simulink model "sp1450WECSminiProject1"  (R2013a)
settings: Solver=ode45  SolverMode=SingleTasking  StartTime=0.0  StopTime=1  RelTol=1e-3
undefined symbols (not defined in the file): D1, J, Lm, Lr, Ls, P, Rr, Rs
libraries: powerlib x8, sdolib x2
settings Model: Creator=Waseem  LastModifiedBy=Sony
settings DataIOCC: SignalLoggingSaveFormat=ModelDataLogs
settings OptimizationCC: BlockReduction=off  BooleanDataType=off
settings DebuggingCC: SaveWithParameterizedLinksMsg=none  SignalResolutionControl=TryResolveAllWithWarning  SolverPrmCheckMsg=none  MultiTaskDSMMsg=warning  MultiTaskCondExecSysMsg=none  StrictBusMsg=None
settings HardwareCC: TargetUnknown=on
settings RTWCC: IncludeERTFirstTime=on

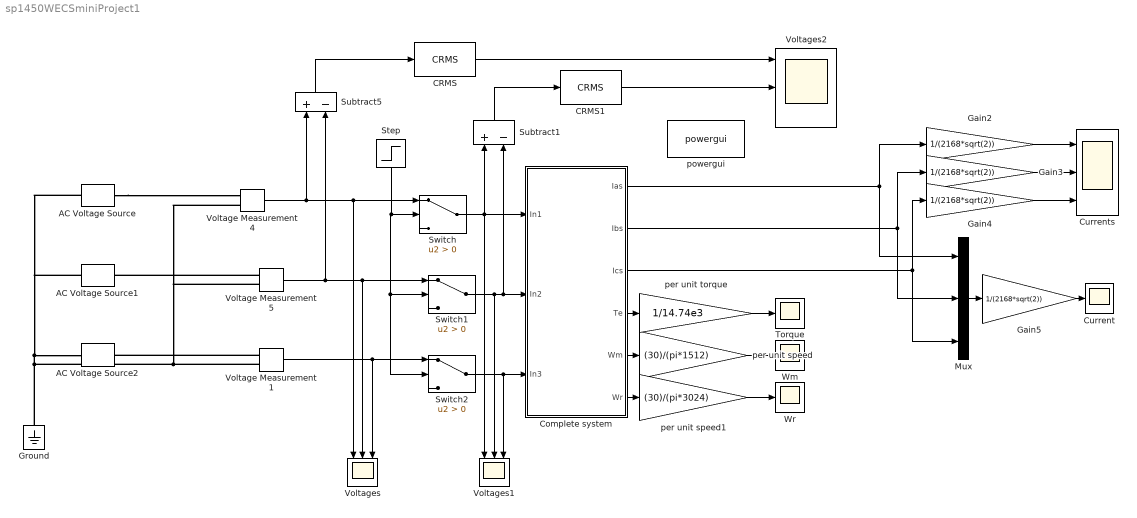
== system sp1450WECSminiProject1 ==
  AC Voltage Source : powerlib/Electrical Sources/AC Voltage Source  Amplitude=563.38264  Phase=0  Frequency=50  SampleTime=0  Measurements=None
  AC Voltage Source1 : powerlib/Electrical Sources/AC Voltage Source  Amplitude=563.38264  Phase=-120  Frequency=50  SampleTime=0  Measurements=None
  AC Voltage Source2 : powerlib/Electrical Sources/AC Voltage Source  Amplitude=563.38264  Phase=-240  Frequency=50  SampleTime=0  Measurements=None
  CRMS : sdolib/RMS Blocks/CRMS
  CRMS1 : sdolib/RMS Blocks/CRMS
  Complete system : Subsystem
  Current : Scope
  Currents : Scope  NumInputPorts=3
      settings: YMin=-5~-5~-5  YMax=5~5~5
  Gain{2..5} (4 alike) : Gain  Gain=1/(2168*sqrt(2))
  Ground : powerlib/Elements/Ground  LConnTagsString=a
  Mux : Mux  Inputs=3
  Step : Step  Time=0  SampleTime=0
  Subtract1 : Sum  Inputs=+-
  Subtract5 : Sum  Inputs=+-
  Switch : Switch  Criteria=u2 > Threshold
  Switch1 : Switch  Criteria=u2 > Threshold
  Switch2 : Switch  Criteria=u2 > Threshold
  Torque : Scope
      settings: YMin=-1.863e-05  YMax=-1.847e-05
  Voltage Measurement1 : powerlib/Measurements/Voltage Measurement  PhasorSimulation=off  OutputType=Complex  PSBequivalent=0
  Voltage Measurement4 : powerlib/Measurements/Voltage Measurement  PhasorSimulation=off  OutputType=Complex  PSBequivalent=0
  Voltage Measurement5 : powerlib/Measurements/Voltage Measurement  PhasorSimulation=off  OutputType=Complex  PSBequivalent=0
  Voltages : Scope  NumInputPorts=3
      settings: YMin=-5~-5~-5  YMax=5~5~5
  Voltages1 : Scope  NumInputPorts=3
      settings: YMin=-5~-5~-5  YMax=5~5~5
  Voltages2 : Scope  NumInputPorts=3
      settings: YMin=-5~-5~-5  YMax=5~5~5  SaveName=ScopeData2
  Wm : Scope
      settings: YMin=37.89  YMax=38.09
  Wr : Scope
      settings: YMin=37.89  YMax=38.09  SaveName=ScopeData3
  per unit speed : Gain  Gain=(30)/(pi*1512)
  per unit speed1 : Gain  Gain=(30)/(pi*3024)
  per unit torque : Gain  Gain=1/14.74e3
  powergui : powerlib/powergui  Priority=1  SimulationMode=Continuous  SolverType=Tustin  SampleTime=50e-6  frequency=50  SPID=on  DisableSnubberDevices=off  DisableRonSwitches=off  DisableVfSwitches=off  SwTol=0  Interpol=off  DisplayEquations=off  frequencyindice=50  Pbase=100e6  ErrMax=1e-4  Iterations=50  UnitsV=kV  UnitsW=MW  FunctionMessages=off  echomessages=off  HookPort=off  EnableUseOfTLC=off  x0status=blocks  RestoreLinks=warning  ResistiveCurrentMeasurement=off  Frange=[0:2:500]  Ylog=off  Xlog=on  ShowGrid=off  save=off  variable=ZData  ZoomFFT=off  StartTime=0.0  cycles=1  DisplayStyle=1  fundamental=60  FreqAxis=off  MaxFrequency=1000  frequencyindicesteady=1  RmsSteady=1  display=off  Ts=0  methode=off
  wires:
  Mux/1 -> Gain5/1
  Voltage Measurement1/1 -> Switch2/1, Voltages/3
  Voltage Measurement5/1 -> Voltages/2, Switch1/1, Subtract5/2
  Complete system/2(Ibs) -> Mux/2, Gain3/1
  Complete system/3(Ics) -> Mux/3, Gain4/1
  Complete system/1(Ias) -> Mux/1, Gain2/1
  Complete system/4(Te) -> per unit torque/1
  Complete system/5(Wm) -> per unit speed/1
  per unit speed/1 -> Wm/1
  Gain2/1 -> Currents/1
  Gain3/1 -> Currents/2
  Gain4/1 -> Currents/3
  Gain5/1 -> Current/1
  Switch/1 -> Subtract1/1, Complete system/1(In1), Voltages1/1
  Switch2/1 -> Complete system/3(In3), Voltages1/3
  Switch1/1 -> Voltages1/2, Complete system/2(In2), Subtract1/2
  Step/1 -> Switch2/2, Switch1/2, Switch/2
  Voltage Measurement4/1 -> Voltages/1, Switch/1, Subtract5/1
  CRMS/1 -> Voltages2/1
  Subtract5/1 -> CRMS/1
  CRMS1/1 -> Voltages2/2
  Subtract1/1 -> CRMS1/1
  per unit torque/1 -> Torque/1
  Complete system/6(Wr) -> per unit speed1/1
  per unit speed1/1 -> Wr/1
  connections:
  Ground/LConn1 -- AC Voltage Source1/LConn1 -- AC Voltage Source/LConn1 -- AC Voltage Source2/LConn1 -- Voltage Measurement5/LConn2 -- Voltage Measurement4/LConn2 -- Voltage Measurement1/LConn2
  AC Voltage Source/RConn1 -- Voltage Measurement4/LConn1
  Voltage Measurement5/LConn1 -- AC Voltage Source1/RConn1
  Voltage Measurement1/LConn1 -- AC Voltage Source2/RConn1

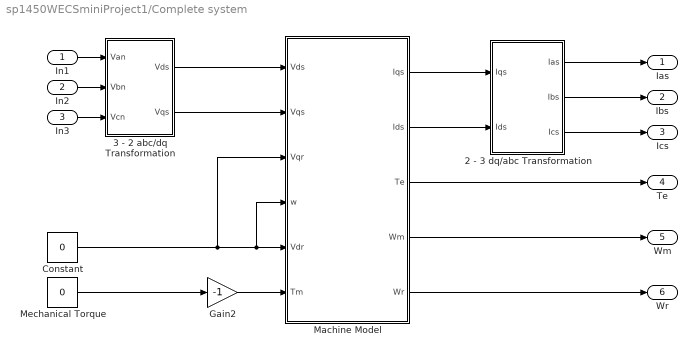
== system sp1450WECSminiProject1/Complete system ==
  In1 : Inport
  In2 : Inport  Port=2
  In3 : Inport  Port=3
  2 - 3 dq/abc Transformation : Subsystem
  3 - 2 abc/dq Transformation : Subsystem
  Constant : Constant  Value=0
  Gain2 : Gain  Gain=-1  ParamDataTypeStr=double
  Machine Model : Subsystem
  Mechanical Torque : Constant  Value=0
  Ias : Outport
  Ibs : Outport  Port=2
  Ics : Outport  Port=3
  Te : Outport  Port=4
  Wm : Outport  Port=5
  Wr : Outport  Port=6
  wires:
  2 - 3 dq/abc Transformation/2(Ibs) -> Ibs/1
  2 - 3 dq/abc Transformation/3(Ics) -> Ics/1
  2 - 3 dq/abc Transformation/1(Ias) -> Ias/1
  Constant/1 -> Machine Model/3(Vqr), Machine Model/4(w), Machine Model/5(Vdr)
  Machine Model/4(Wm) -> Wm/1
  Machine Model/1(Iqs) -> 2 - 3 dq/abc Transformation/1(Iqs)
  3 - 2 abc/dq Transformation/1(Vds) -> Machine Model/1(Vds)
  Machine Model/2(Ids) -> 2 - 3 dq/abc Transformation/2(Ids)
  3 - 2 abc/dq Transformation/2(Vqs) -> Machine Model/2("Vqs ")
  Gain2/1 -> Machine Model/6(Tm)
  Machine Model/3(Te) -> Te/1
  Mechanical Torque/1 -> Gain2/1
  In2/1 -> 3 - 2 abc/dq Transformation/2(Vbn)
  In1/1 -> 3 - 2 abc/dq Transformation/1(Van)
  In3/1 -> 3 - 2 abc/dq Transformation/3(Vcn)
  Machine Model/5(Wr) -> Wr/1

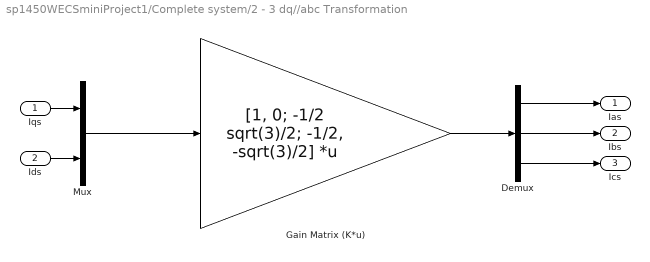
== system sp1450WECSminiProject1/Complete system/2 - 3 dq//abc Transformation ==
  Iqs : Inport
  Ids : Inport  Port=2
  Demux : Demux  Outputs=3
  Gain Matrix (K*u) : Gain  Gain=[1, 0; -1/2 sqrt(3)/2; -1/2, -sqrt(3)/2]  Multiplication=Matrix(K*u)
  Mux : Mux  Inputs=2
  Ias : Outport
  Ibs : Outport  Port=2
  Ics : Outport  Port=3
  wires:
  Mux/1 -> Gain Matrix (K*u)/1
  Gain Matrix (K*u)/1 -> Demux/1
  Demux/2 -> Ibs/1
  Demux/1 -> Ias/1
  Demux/3 -> Ics/1
  Iqs/1 -> Mux/1
  Ids/1 -> Mux/2

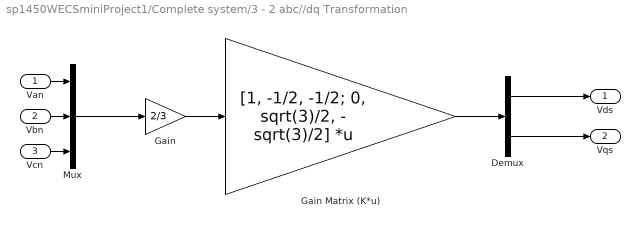
== system sp1450WECSminiProject1/Complete system/3 - 2 abc//dq Transformation ==
  Van : Inport
  Vbn : Inport  Port=2
  Vcn : Inport  Port=3
  Demux : Demux  Outputs=2
  Gain : Gain  Gain=2/3
  Gain Matrix (K*u) : Gain  Gain=[1, -1/2, -1/2; 0, sqrt(3)/2, - sqrt(3)/2]  Multiplication=Matrix(K*u)
  Mux : Mux  Inputs=3
  Vds : Outport
  Vqs : Outport  Port=2
  wires:
  Vcn/1 -> Mux/3
  Vbn/1 -> Mux/2
  Van/1 -> Mux/1
  Gain/1 -> Gain Matrix (K*u)/1
  Gain Matrix (K*u)/1 -> Demux/1
  Mux/1 -> Gain/1
  Demux/1 -> Vds/1
  Demux/2 -> Vqs/1

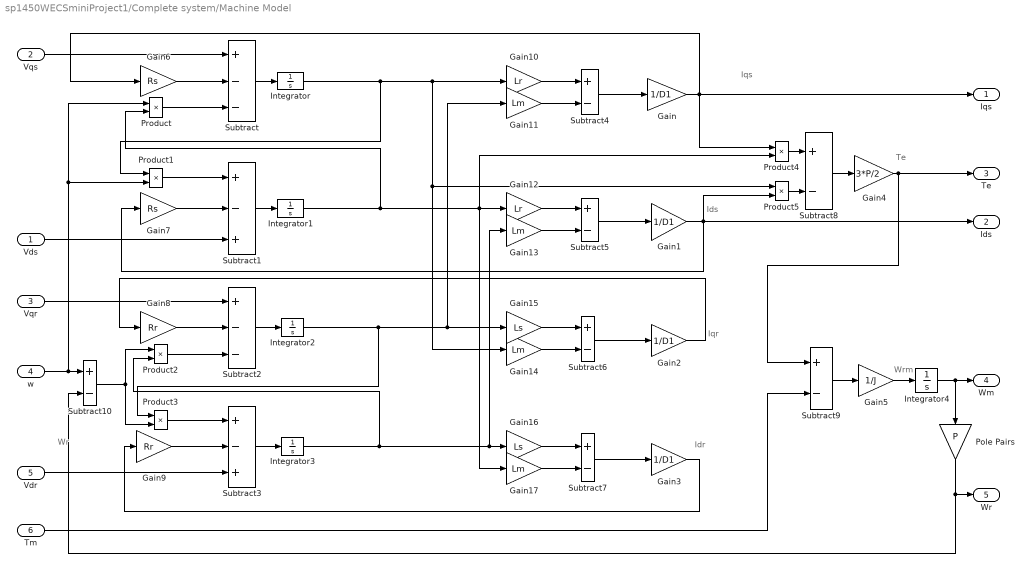
== system sp1450WECSminiProject1/Complete system/Machine Model ==
  note: Idr
  note: Iqr
  note: Te
  note: Ids
  note: Iqs
  note: Wrm
  note: Wr
  Vds : Inport
  "Vqs " : Inport  Port=2
  Vqr : Inport  Port=3
  w : Inport  Port=4
  Vdr : Inport  Port=5
  Tm : Inport  Port=6
  Gain{,1..3} (4 alike) : Gain  Gain=1/D1
  Gain10 : Gain  Gain=Lr
  Gain{11,13..14,17} (4 alike) : Gain  Gain=Lm
  Gain12 : Gain  Gain=Lr
  Gain15 : Gain  Gain=Ls
  Gain16 : Gain  Gain=Ls
  Gain4 : Gain  Gain=3*P/2
  Gain5 : Gain  Gain=1/J
  Gain6 : Gain  Gain=Rs
  Gain7 : Gain  Gain=Rs
  Gain8 : Gain  Gain=Rr
  Gain9 : Gain  Gain=Rr
  Integrator{,1..3} (4 alike) : Integrator
  Integrator4 : Integrator  InitialCondition=151.843644924  IgnoreLimit=on
  Pole Pairs : Gain  Gain=P
  Product{,1..5} (6 alike) : Product
  Subtract : Sum  Inputs=+--
  Subtract1 : Sum  Inputs=+-+
  Subtract{4..10} (7 alike) : Sum  Inputs=+-
  Subtract2 : Sum  Inputs=+--
  Subtract3 : Sum  Inputs=+-+
  Iqs : Outport
  Ids : Outport  Port=2
  Te : Outport  Port=3
  Wm : Outport  Port=4
  Wr : Outport  Port=5
  wires:
  Subtract/1 -> Integrator/1
  Integrator/1 -> Gain10/1, Product5/1, Gain14/1, Product1/1
  Subtract1/1 -> Integrator1/1
  Subtract2/1 -> Integrator2/1
  Subtract3/1 -> Integrator3/1
  Subtract4/1 -> Gain/1
  Subtract5/1 -> Gain1/1
  Subtract6/1 -> Gain2/1
  Subtract7/1 -> Gain3/1
  Subtract8/1 -> Gain4/1
  Subtract9/1 -> Gain5/1
  Product4/1 -> Subtract8/1
  Gain/1 -> Product4/1, Iqs/1, Gain6/1
  Gain10/1 -> Subtract4/1
  Gain11/1 -> Subtract4/2
  Gain6/1 -> Subtract/2
  Product/1 -> Subtract/3
  Product1/1 -> Subtract1/1
  Gain7/1 -> Subtract1/2
  w/1 -> Product/1, Product1/2, Subtract10/1
  Gain12/1 -> Subtract5/1
  Gain13/1 -> Subtract5/2
  Integrator1/1 -> Gain17/1, Product4/2, Gain12/1, Product/2
  Gain1/1 -> Gain7/1, Ids/1, Product5/2
  Product5/1 -> Subtract8/2
  Gain4/1 -> Te/1, Subtract9/1
  Gain8/1 -> Subtract2/2
  Product2/1 -> Subtract2/3
  Vqr/1 -> Subtract2/1
  Gain14/1 -> Subtract6/2
  Gain15/1 -> Subtract6/1
  Integrator2/1 -> Gain11/1, Gain15/1, Product3/1
  Gain2/1 -> Gain8/1
  Subtract10/1 -> Product3/2, Product2/1
  Product3/1 -> Subtract3/1
  Gain9/1 -> Subtract3/2
  Integrator3/1 -> Product2/2, Gain13/1, Gain16/1
  Gain16/1 -> Subtract7/1
  Gain17/1 -> Subtract7/2
  Gain3/1 -> Gain9/1
  Gain5/1 -> Integrator4/1
  Integrator4/1 -> Pole Pairs/1, Wm/1
  Pole Pairs/1 -> Wr/1, Subtract10/2
  Tm/1 -> Subtract9/2
  Vdr/1 -> Subtract3/3
  Vds/1 -> Subtract1/3
  "Vqs "/1 -> Subtract/1
